simulink subsystem "cvs_calculations"  (R2020b)
settings: Solver=VariableStepAuto  StartTime=0.0  StopTime=10.0  RelTol=1e-3
values from neighbouring files (symbols this model uses):
  P_default = [105.55 4 15 6]    [model_workspace.mat]
settings Model: Creator=RH  LastModifiedBy=fonck

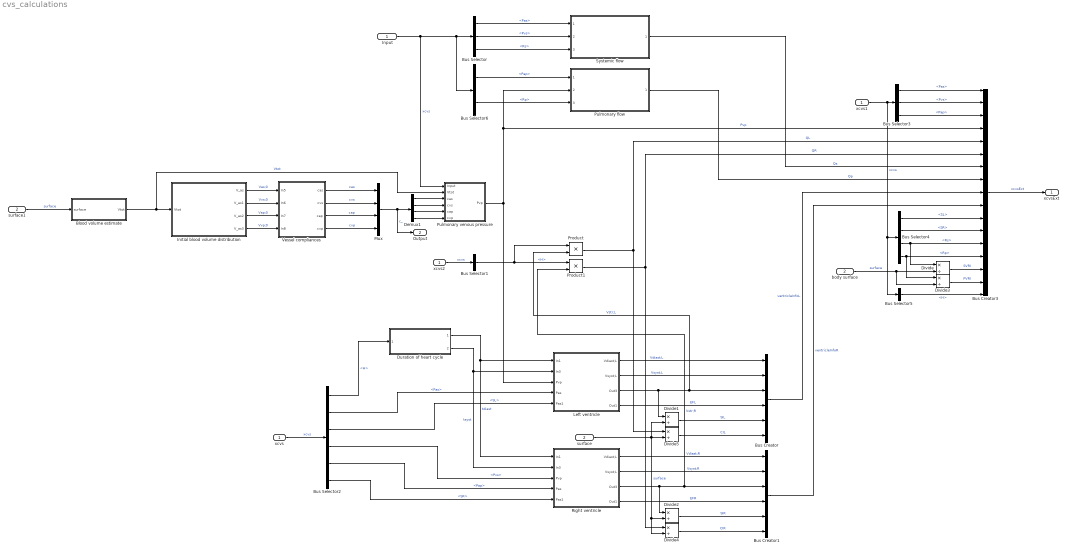
== system cvs_calculations ==
  Input : Inport  OutDataTypeStr=Bus: CardioVascularState
  body surface : Inport  Port=2  Unit=m^2
  Blood volume estimate : Subsystem  TreatAsAtomicUnit=on
  Bus Creator : BusCreator  Inputs=6  OutDataTypeStr=Bus: ventricleInfo
      settings: InheritFromInputs=off
  Bus Creator1 : BusCreator  Inputs=6  OutDataTypeStr=Bus: ventricleInfo
      settings: InheritFromInputs=off
  Bus Creator3 : BusCreator  Inputs=17  OutDataTypeStr=Bus: CardioVascularStateExtended
      settings: InheritFromInputs=off
  Bus Selector : BusSelector  OutputSignals=Pas,Pvs,Rs
  Bus Selector1 : BusSelector  OutputSignals=H
  Bus Selector2 : BusSelector  OutputSignals=H,Pas,SL,Pvs,Pap,SR
  Bus Selector3 : BusSelector  OutputSignals=Pas,Pvs,Pap
  Bus Selector4 : BusSelector  OutputSignals=SL,SR,Rs,Rp
  Bus Selector5 : BusSelector  OutputSignals=H
  Bus Selector6 : BusSelector  OutputSignals=Pap,Rp
  Demux1 : Demux
  Divide{,1..5} (6 alike) : Product  Inputs=*/
  Duration of heart cycle : Subsystem  TreatAsAtomicUnit=on  ReferencedSubsystem=cvrs_heart_cycle
  Initial blood volume distribution : Subsystem  TreatAsAtomicUnit=on
  Left ventricle : Subsystem
  Mux : Mux
  Product : Product
  Product1 : Product
  Pulmonary flow : Subsystem  ReferencedSubsystem=blood_compartment_flow_2
  Pulmonary venous pressure : Subsystem
  Right ventricle : Subsystem
  Systemic flow : Subsystem  ReferencedSubsystem=blood_compartment_flow_2
  Vessel compliances : Subsystem  TreatAsAtomicUnit=on
  surface : InportShadow  Port=2  Unit=m^2
  surface1 : InportShadow  Port=2  Unit=m^2
  xcvs : InportShadow  OutDataTypeStr=Bus: CardioVascularState
  xcvs1 : InportShadow  OutDataTypeStr=Bus: CardioVascularState
  xcvs2 : InportShadow  OutDataTypeStr=Bus: CardioVascularState
  xcvsExt : Outport  OutDataTypeStr=Bus: CardioVascularStateExtended
  Output : Outport  Port=2  Unit=L/mmHg  PortDimensions=4
  wires:
  Mux/1 -> Output/1, Demux1/1  "c_"
  Demux1/3 -> Pulmonary venous pressure/5(cap)
  Right ventricle/2(Vsyst;L) -> Bus Creator1/2  "Vsyst;R"
  Left ventricle/4(Out1) -> Bus Creator/4  "EFL"
  Bus Selector4/1 -> Bus Creator3/11  "<SL>"
  Right ventricle/4(Out1) -> Bus Creator1/4  "EFR"
  Bus Selector/3 -> Systemic flow/3  "<Rs>"
  Right ventricle/3(Out3) -> Product1/2, Bus Creator1/3, Divide2/1  "Vstr;R"
  Divide4/1 -> Bus Creator1/6  "CIR"
  Bus Selector/2 -> Systemic flow/2  "<Pvs>"
  Bus Creator/1 -> Bus Creator3/9  "ventricleInfoL"
  Duration of heart cycle/2 -> Left ventricle/2(In3), Right ventricle/2(In3)  "tsyst"
  Divide1/1 -> Bus Creator/5  "SIL"
  Bus Selector2/4 -> Right ventricle/3(Pvp)  "<Pvs>"
  Bus Selector3/3 -> Bus Creator3/3  "<Pap>"
  Product/1 -> Bus Creator3/5, Divide5/1  "QL"
  Demux1/1 -> Pulmonary venous pressure/3(cas)
  Duration of heart cycle/1 -> Left ventricle/1(In1), Right ventricle/1(In1)  "tdiast"
  Pulmonary venous pressure/1(Pvp) -> Left ventricle/3(Pvp), Bus Creator3/4, Pulmonary flow/2  "Pvp"
  xcvs1/1 -> Bus Selector3/1, Bus Selector4/1, Bus Selector5/1  "xcvs"
  Bus Selector1/1 -> Product1/1, Product/1  "<H>"
  Bus Creator3/1 -> xcvsExt/1  "xcvsExt"
  Demux1/2 -> Pulmonary venous pressure/4(cvs)
  Divide2/1 -> Bus Creator1/5  "SIR"
  Left ventricle/3(Out3) -> Divide1/1, Bus Creator/3, Product/2  "Vstr;L"
  Bus Selector6/2 -> Pulmonary flow/3  "<Rp>"
  Bus Selector2/2 -> Left ventricle/4(Pas)  "<Pas>"
  Bus Selector5/1 -> Bus Creator3/17  "<H>"
  Bus Selector3/1 -> Bus Creator3/1  "<Pas>"
  Pulmonary flow/1 -> Bus Creator3/8  "Qp"
  Bus Selector2/3 -> Left ventricle/5(Pas1)  "<SL>"
  Divide5/1 -> Bus Creator/6  "CIL"
  Product1/1 -> Bus Creator3/6, Divide4/1  "QR"
  Input/1 -> Bus Selector6/1, Bus Selector/1, Pulmonary venous pressure/1(Input)  "xcvs"
  Bus Selector2/1 -> Duration of heart cycle/1  "<H>"
  Bus Selector/1 -> Systemic flow/1  "<Pas>"
  Bus Selector6/1 -> Pulmonary flow/1  "<Pap>"
  xcvs/1 -> Bus Selector2/1  "xcvs"
  Left ventricle/1(Vdiast;L) -> Bus Creator/1  "Vdiast;L"
  Bus Selector2/6 -> Right ventricle/5(Pas1)  "<SR>"
  Bus Selector4/2 -> Bus Creator3/12  "<SR>"
  Bus Creator1/1 -> Bus Creator3/10  "ventricleInfoR"
  Bus Selector3/2 -> Bus Creator3/2  "<Pvs>"
  Left ventricle/2(Vsyst;L) -> Bus Creator/2  "Vsyst;L"
  Bus Selector4/4 -> Bus Creator3/14, Divide3/1  "<Rp>"
  Bus Selector4/3 -> Bus Creator3/13, Divide/1  "<Rs>"
  Right ventricle/1(Vdiast;L) -> Bus Creator1/1  "Vdiast;R"
  Divide3/1 -> Bus Creator3/16  "PVRI"
  Divide/1 -> Bus Creator3/15  "SVRI"
  surface/1 -> Divide5/2, Divide2/2, Divide4/2, Divide1/2  "surface"
  Systemic flow/1 -> Bus Creator3/7  "Qs"
  Bus Selector2/5 -> Right ventricle/4(Pas)  "<Pap>"
  body surface/1 -> Divide3/2, Divide/2  "surface"
  Demux1/4 -> Pulmonary venous pressure/6(cvp)
  xcvs2/1 -> Bus Selector1/1  "xcvs"
  Initial blood volume distribution/2(V_as1) -> Vessel compliances/2(In6)  "Vvs;0"
  Vessel compliances/3(cap) -> Mux/3  "cap"
  Initial blood volume distribution/1(V_as) -> Vessel compliances/1(In5)  "Vas;0"
  Vessel compliances/4(cvp) -> Mux/4  "cvp"
  Vessel compliances/2(cvs) -> Mux/2  "cvs"
  Vessel compliances/1(cas) -> Mux/1  "cas"
  Initial blood volume distribution/3(V_as2) -> Vessel compliances/3(In7)  "Vap;0"
  Initial blood volume distribution/4(V_as3) -> Vessel compliances/4(In8)  "Vvp;0"
  surface1/1 -> Blood volume estimate/1(surface)  "surface"
  Blood volume estimate/1(Vtot) -> Pulmonary venous pressure/2(Vtot), Initial blood volume distribution/1(Vtot)  "Vtot"

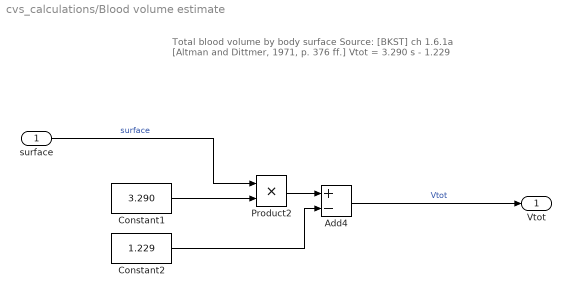
== system cvs_calculations/Blood volume estimate ==
  note: Total blood volume by body surface
      | Source: [BKST] ch 1.6.1a [Altman and Dittmer, 1971, p. 376 ff.]
      | Vtot = 3.290 s - 1.229
  surface : Inport  Unit=m^2
  Add4 : Sum  Inputs=+-
  Constant1 : Constant  Value=3.290
  Constant2 : Constant  Value=1.229
  Product2 : Product
  Vtot : Outport  Unit=L
  wires:
  surface/1 -> Product2/1  "surface"
  Add4/1 -> Vtot/1  "Vtot"
  Constant1/1 -> Product2/2
  Product2/1 -> Add4/1
  Constant2/1 -> Add4/2

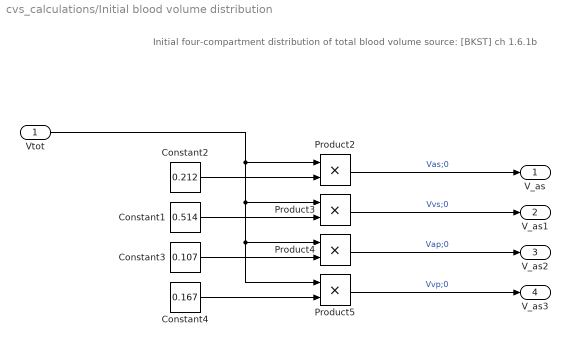
== system cvs_calculations/Initial blood volume distribution ==
  note: Initial four-compartment distribution of total blood volume
      | source: [BKST] ch 1.6.1b
  Vtot : Inport  Unit=L
  Constant1 : Constant  Value=0.514
  Constant2 : Constant  Value=0.212
  Constant3 : Constant  Value=0.107
  Constant4 : Constant  Value=0.167
  Product{2..5} (4 alike) : Product
  V_as : Outport  Unit=L
  V_as1 : Outport  Port=2  Unit=L
  V_as2 : Outport  Port=3  Unit=L
  V_as3 : Outport  Port=4  Unit=L
  wires:
  Product5/1 -> V_as3/1  "Vvp;0"
  Product4/1 -> V_as2/1  "Vap;0"
  Product3/1 -> V_as1/1  "Vvs;0"
  Constant2/1 -> Product2/2
  Constant4/1 -> Product5/2
  Vtot/1 -> Product5/1, Product4/1, Product3/1, Product2/1
  Product2/1 -> V_as/1  "Vas;0"
  Constant3/1 -> Product4/2
  Constant1/1 -> Product3/2

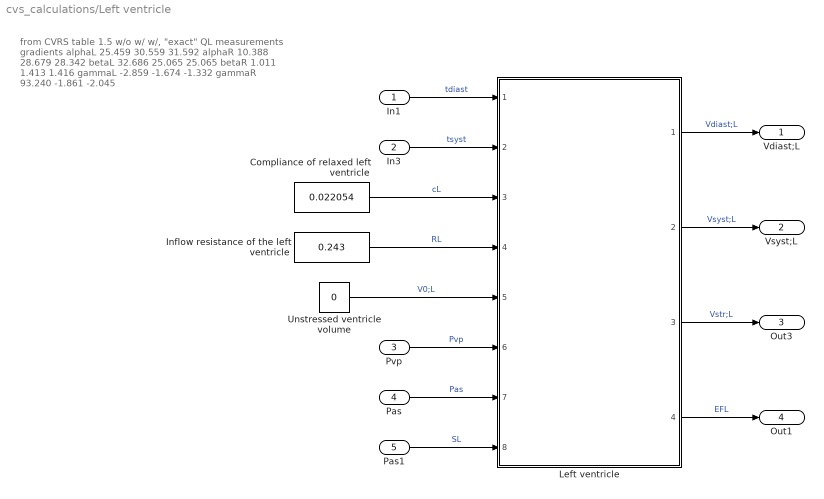
== system cvs_calculations/Left ventricle ==
  note: from CVRS table 1.5
      | w/o w/ w/, "exact"
      | QL measurements gradients
      |
      | alphaL 25.459 30.559 31.592
      | alphaR 10.388 28.679 28.342
      | betaL 32.686 25.065 25.065
      | betaR 1.011 1.413 1.416
      | gammaL -2.859 -1.674 -1.332
      | gammaR 93.240 -1.861 -2.045
  In1 : Inport  Unit=s
  In3 : Inport  Port=2  Unit=s
  Pvp : Inport  Port=3  Unit=mmHg
  Pas : Inport  Port=4  Unit=mmHg
  Pas1 : Inport  Port=5  Unit=mmHg
  Compliance of relaxed left ventricle : Constant  Value=0.022054
  Inflow resistance of the left ventricle : Constant  Value=0.243
  Left ventricle : Subsystem  ReferencedSubsystem=cvrs_ventricle
  Unstressed ventricle volume : Constant  Value=0
  Vdiast;L : Outport  Unit=liter
  Vsyst;L : Outport  Port=2  Unit=liter
  Out3 : Outport  Port=3  Unit=liter
  Out1 : Outport  Port=4  Unit=1
  wires:
  Pas1/1 -> Left ventricle/8  "SL"
  Left ventricle/4 -> Out1/1  "EFL"
  Left ventricle/2 -> Vsyst;L/1  "Vsyst;L"
  Pvp/1 -> Left ventricle/6  "Pvp"
  In1/1 -> Left ventricle/1  "tdiast"
  Left ventricle/1 -> Vdiast;L/1  "Vdiast;L"
  Left ventricle/3 -> Out3/1  "Vstr;L"
  In3/1 -> Left ventricle/2  "tsyst"
  Inflow resistance of the left ventricle/1 -> Left ventricle/4  "RL"
  Pas/1 -> Left ventricle/7  "Pas"
  Compliance of relaxed left ventricle/1 -> Left ventricle/3  "cL"
  Unstressed ventricle volume/1 -> Left ventricle/5  "V0;L"

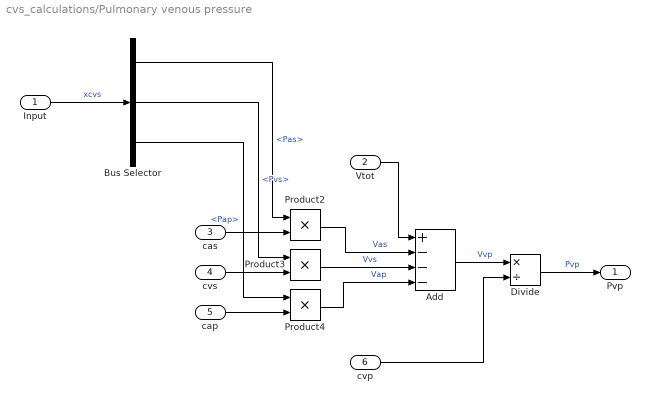
== system cvs_calculations/Pulmonary venous pressure ==
  Input : Inport  OutDataTypeStr=Bus: CardioVascularState
  Vtot : Inport  Port=2
  cas : Inport  Port=3
  cvs : Inport  Port=4
  cap : Inport  Port=5
  cvp : Inport  Port=6
  Add : Sum  Inputs=+---
  Bus Selector : BusSelector  OutputSignals=Pas,Pvs,Pap
  Divide : Product  Inputs=*/
  Product2 : Product
  Product3 : Product
  Product4 : Product
  Pvp : Outport  Unit=mmHg
  wires:
  Input/1 -> Bus Selector/1  "xcvs"
  Divide/1 -> Pvp/1  "Pvp"
  cap/1 -> Product4/2
  Vtot/1 -> Add/1
  cas/1 -> Product2/2
  cvs/1 -> Product3/2
  Product2/1 -> Add/2  "Vas"
  Bus Selector/2 -> Product3/1  "<Pvs>"
  Product3/1 -> Add/3  "Vvs"
  Bus Selector/3 -> Product4/1  "<Pap>"
  Add/1 -> Divide/1  "Vvp"
  Bus Selector/1 -> Product2/1  "<Pas>"
  cvp/1 -> Divide/2
  Product4/1 -> Add/4  "Vap"

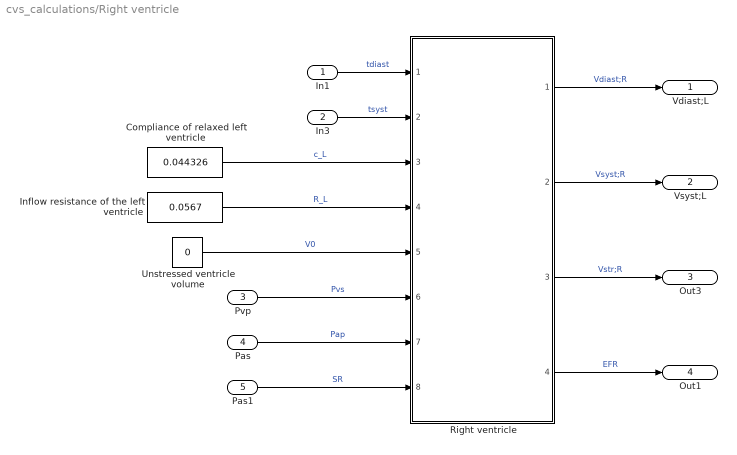
== system cvs_calculations/Right ventricle ==
  In1 : Inport  Unit=s
  In3 : Inport  Port=2  Unit=s
  Pvp : Inport  Port=3  Unit=mmHg
  Pas : Inport  Port=4  Unit=mmHg
  Pas1 : Inport  Port=5  Unit=mmHg
  Compliance of relaxed left ventricle : Constant  Value=0.044326
  Inflow resistance of the left ventricle : Constant  Value=0.0567
  Right ventricle : Subsystem  ReferencedSubsystem=cvrs_ventricle
  Unstressed ventricle volume : Constant  Value=0
  Vdiast;L : Outport  Unit=liter
  Vsyst;L : Outport  Port=2  Unit=liter
  Out3 : Outport  Port=3  Unit=liter
  Out1 : Outport  Port=4  Unit=1
  wires:
  Pas1/1 -> Right ventricle/8  "SR"
  Right ventricle/4 -> Out1/1  "EFR"
  Unstressed ventricle volume/1 -> Right ventricle/5  "V0"
  Compliance of relaxed left ventricle/1 -> Right ventricle/3  "c_L"
  Pas/1 -> Right ventricle/7  "Pap"
  Inflow resistance of the left ventricle/1 -> Right ventricle/4  "R_L"
  In3/1 -> Right ventricle/2  "tsyst"
  Right ventricle/3 -> Out3/1  "Vstr;R"
  Right ventricle/1 -> Vdiast;L/1  "Vdiast;R"
  In1/1 -> Right ventricle/1  "tdiast"
  Pvp/1 -> Right ventricle/6  "Pvs"
  Right ventricle/2 -> Vsyst;L/1  "Vsyst;R"

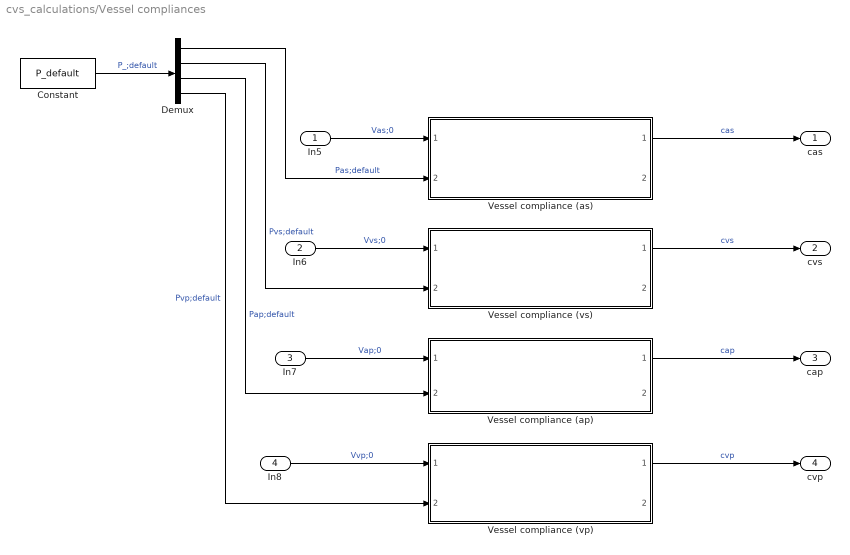
== system cvs_calculations/Vessel compliances ==
  In5 : Inport  Unit=L
  In6 : Inport  Port=2  Unit=L
  In7 : Inport  Port=3  Unit=L
  In8 : Inport  Port=4  Unit=L
  Constant : Constant  Value=P_default
  Demux : Demux
  Vessel compliance (ap) : Subsystem  ReferencedSubsystem=vessel_compliance
  Vessel compliance (as) : Subsystem  ReferencedSubsystem=vessel_compliance
  Vessel compliance (vp) : Subsystem  ReferencedSubsystem=vessel_compliance
  Vessel compliance (vs) : Subsystem  ReferencedSubsystem=vessel_compliance
  cas : Outport  Unit=L/mmHg
  cvs : Outport  Port=2  Unit=L/mmHg
  cap : Outport  Port=3  Unit=L/mmHg
  cvp : Outport  Port=4  Unit=L/mmHg
  wires:
  Constant/1 -> Demux/1  "P_;default"
  Vessel compliance (vs)/1 -> cvs/1  "cvs"
  Vessel compliance (as)/1 -> cas/1  "cas"
  In8/1 -> Vessel compliance (vp)/1  "Vvp;0"
  Vessel compliance (ap)/1 -> cap/1  "cap"
  Demux/1 -> Vessel compliance (as)/2  "Pas;default"
  In6/1 -> Vessel compliance (vs)/1  "Vvs;0"
  Demux/4 -> Vessel compliance (vp)/2  "Pvp;default"
  Vessel compliance (vp)/1 -> cvp/1  "cvp"
  Demux/2 -> Vessel compliance (vs)/2  "Pvs;default"
  In7/1 -> Vessel compliance (ap)/1  "Vap;0"
  In5/1 -> Vessel compliance (as)/1  "Vas;0"
  Demux/3 -> Vessel compliance (ap)/2  "Pap;default"
